simulink model "model"  (R2016a)
settings: Solver=VariableStepAuto  StartTime=0.0  StopTime=50  RelTol=1e-3
undefined symbols (not defined in the file or in its folder): params
settings Model: Creator=user  LastModifiedBy=user

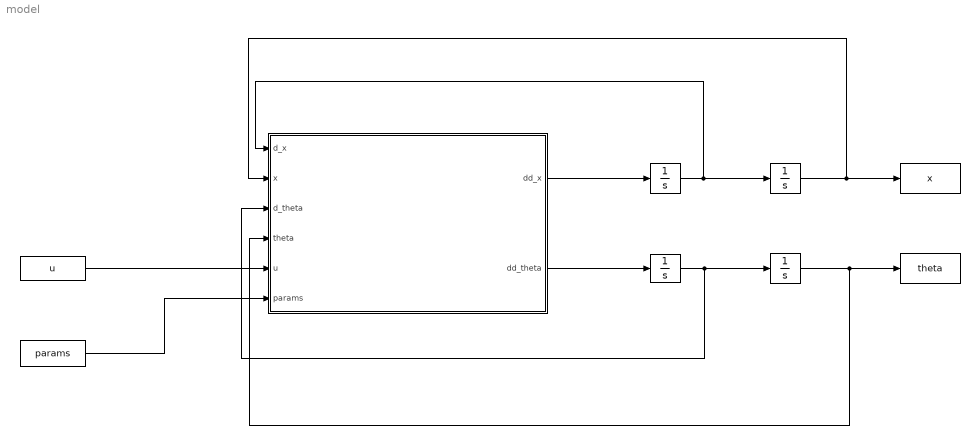
== system model ==
   {,,,} (4 alike) : Integrator
  " " : FromWorkspace  VariableName=u  SampleTime=0
  " " : Constant  Value=params  OutDataTypeStr=Bus: params_bus
  " " : ToWorkspace  VariableName=x  SaveFormat=Timeseries  SampleTime=-1
  " " : ToWorkspace  VariableName=theta  SaveFormat=Timeseries  SampleTime=-1
  " " : MATLAB Function  TreatAsAtomicUnit=on
  wires:
  " "/1(dd_x) -> " "/1
  " "/2(dd_theta) -> " "/1
  " "/1 -> " "/1, " "/1(d_x)
  " "/1 -> " "/3(d_theta), " "/1
  " "/1 -> " "/5(u)
  " "/1 -> " "/6(params)
  " "/1 -> " "/2(x), " "/1
  " "/1 -> " "/4(theta), " "/1

== matlab function model/  ==
  data: d_x input; x input; d_theta input; theta input; u input; dd_x output; params input; dd_theta output
function [dd_x, dd_theta] = fcn(d_x, x, d_theta, theta, u, params)
    dd_x = params.l * (d_theta)^2 - (params.k*x)/params.m + params.g*cos(theta) - params.zeta * d_x;
    dd_theta = (-params.g*sin(theta))/params.l - (2 * d_x * d_theta)/params.l - params.zeta * d_theta + u/(params.m * params.l^2);
y = u;
